simulink model "Main"  (R2020a)
settings: Solver=VariableStepAuto  StartTime=0.0  StopTime=param.taskDuration  RelTol=1e-3
InitFcn:
  | Init
StopFcn:
  | StopSim
undefined symbols (not defined in the file or in its folder): data, DiscIntNeverNeededParam, param
settings Model: Creator=dell  LastModifiedBy=yupeng
settings DebuggingCC: SFMachineParentedDataDiag=error

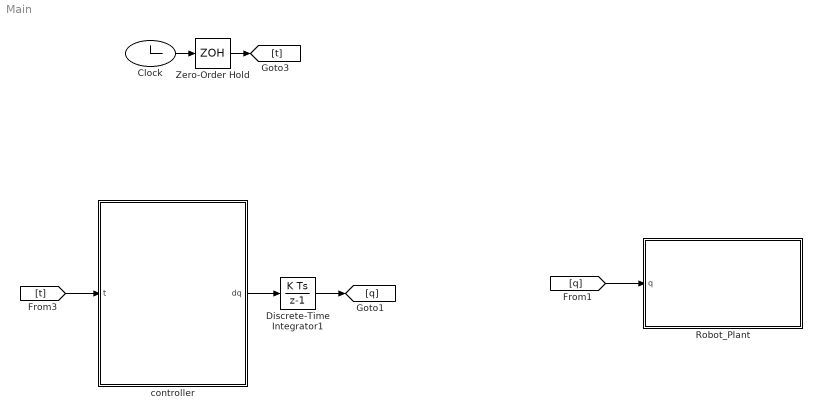
== system Main ==
  Clock : Clock
  Discrete-Time Integrator1 : DiscreteIntegrator  InitialCondition=data.inputAngle(:,1)  SampleTime=-1  ICPrevOutput=DiscIntNeverNeededParam  ICPrevScaledInput=DiscIntNeverNeededParam
  Robot_Plant : MATLAB Function  TreatAsAtomicUnit=on
  Zero-Order Hold : ZeroOrderHold  SampleTime=param.step
  controller : MATLAB Function  TreatAsAtomicUnit=on
  wires:
  Zero-Order Hold/1 -> [t]
  Clock/1 -> Zero-Order Hold/1
  Discrete-Time Integrator1/1 -> [q]
  [q] -> Robot_Plant/1(q)
  [t] -> controller/1(t)
  controller/1(dq) -> Discrete-Time Integrator1/1

== matlab function Main/Robot_Plant ==
  data: q input
function fcn(q)
coder.extrinsic('RobotPlant');

RobotPlant(q);

end

== matlab function Main/controller ==
  data: t input; dq output
function dq  = fcn(t)
coder.extrinsic('Algorithm');
dq = zeros(6,1);
dJHat = zeros(3,7);

output = double(Algorithm());
dq = output(1,1:6)';
% dJHat = output(2:4,1:7);

end
